simulink model "teleop_sim"  (R2019a)
settings: Solver=VariableStepAuto  StartTime=0.0  StopTime=10  MaxStep=dt  RelTol=1e-3
model workspace: external: MATLAB File .\teleop_sim_setup.m (data not in the file)
undefined symbols (not defined in the file): A_v, b, d_T, derivative_phases, epsilon, f_0, K_d, K_p, m, Ts, v_0, w_v, x_0
settings Model: Creator=Shane  LastModifiedBy=17stf1
settings DataIOCC: ReturnWorkspaceOutputs=off
settings DebuggingCC: PregeneratedLibrarySubsystemCodeDiagnostic=none  StrictBusMsg=WarnOnBusTreatedAsVector  ArithmeticOperatorsInVariantConditions=warning
settings SFSimCC: SimUseLocalCustomCode=off
settings RTWCC: RTWUseLocalCustomCode=off

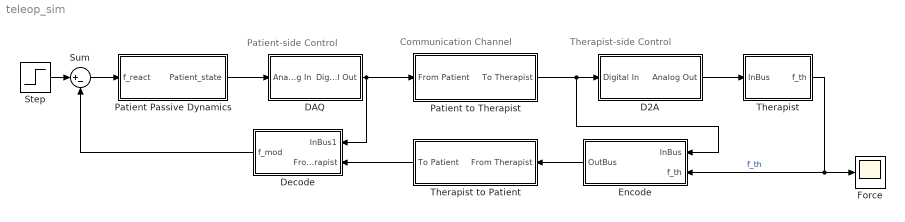
== system teleop_sim ==
  note: Patient-side Control
  note: Therapist-side Control
  note: Communication Channel
  D2A : Subsystem
  DAQ : Subsystem
  Decode : Subsystem
  Encode : Subsystem
  Force : Scope
  Patient Passive Dynamics : Subsystem
  Patient to Therapist : Subsystem
  Step : Step  After=0  SampleTime=0
  Sum : Sum  Inputs=|+-
  Therapist : Subsystem
  Therapist to Patient : Subsystem
  wires:
  Sum/1 -> Patient Passive Dynamics/1(f_react)
  Patient Passive Dynamics/1(Patient_state) -> DAQ/1(Analog In)
  Step/1 -> Sum/1
  Therapist/1(f_th) -> Force/1, Encode/2(f_th)  "f_th"
  Patient to Therapist/1(To Therapist) -> D2A/1(Digital In), Encode/1(InBus)
  Encode/1(OutBus) -> Therapist to Patient/1(From Therapist)
  Therapist to Patient/1(To Patient) -> Decode/2(FromTherapist)
  Decode/1(f_mod) -> Sum/2
  DAQ/1(Digital Out) -> Decode/1(InBus1), Patient to Therapist/1(From Patient)
  D2A/1(Analog Out) -> Therapist/1(InBus)

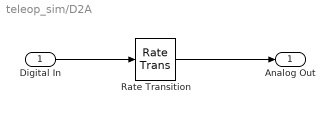
== system teleop_sim/D2A ==
  Digital In : Inport
  Rate Transition : RateTransition
  Analog Out : Outport
  wires:
  Digital In/1 -> Rate Transition/1
  Rate Transition/1 -> Analog Out/1

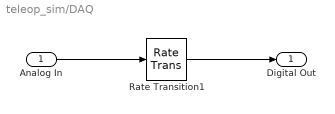
== system teleop_sim/DAQ ==
  Analog In : Inport
  Rate Transition1 : RateTransition  OutPortSampleTime=Ts
  Digital Out : Outport
  wires:
  Analog In/1 -> Rate Transition1/1
  Rate Transition1/1 -> Digital Out/1

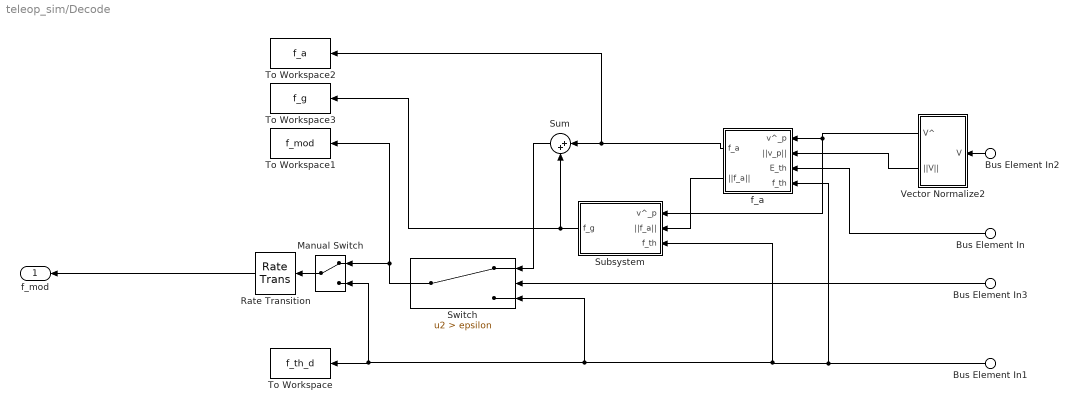
== system teleop_sim/Decode ==
  Bus Element In2 : Inport  PortName=InBus1  Element=v_p
  Bus Element In : Inport  Port=2  PortName=FromTherapist  Element=E_th
  Bus Element In1 : Inport  Port=2  PortName=FromTherapist  Element=f_th
  Bus Element In3 : Inport  Port=2  PortName=FromTherapist  Element=v_mag
  Manual Switch : ManualSwitch
  Rate Transition : RateTransition
  Subsystem : Subsystem
  Sum : Sum  Inputs=|++
  Switch : Switch  Criteria=u2 > Threshold  Threshold=epsilon
  To Workspace : ToWorkspace  VariableName=f_th_d  SaveFormat=Structure With Time  SampleTime=-1
  To Workspace1 : ToWorkspace  VariableName=f_mod  SaveFormat=Structure With Time  SampleTime=-1
  To Workspace2 : ToWorkspace  VariableName=f_a  SaveFormat=Structure With Time  SampleTime=-1
  To Workspace3 : ToWorkspace  VariableName=f_g  SaveFormat=Structure With Time  SampleTime=-1
  Vector Normalize2 : Subsystem  mask{min_magnitude=epsilon}
      mask prompts: min_magnitude "Minimum magnitude:"
  f_a : Subsystem
  f_mod : Outport
  wires:
  Sum/1 -> Switch/1
  Bus Element In2/1 -> Vector Normalize2/1(V)
  Vector Normalize2/1(V^) -> f_a/1(v^_p), Subsystem/1(v^_p)
  Manual Switch/1 -> Rate Transition/1
  Bus Element In1/1 -> f_a/4(f_th), Subsystem/3(f_th), Manual Switch/2, To Workspace/1, Switch/3
  Rate Transition/1 -> f_mod/1
  Subsystem/1(f_g) -> Sum/2, To Workspace3/1
  Bus Element In3/1 -> Switch/2
  Switch/1 -> Manual Switch/1, To Workspace1/1
  f_a/1(f_a) -> To Workspace2/1, Sum/1
  Vector Normalize2/2(||V||) -> f_a/2(||v_p||)
  Bus Element In/1 -> f_a/3(E_th)
  f_a/2(||f_a||) -> Subsystem/2(||f_a||)

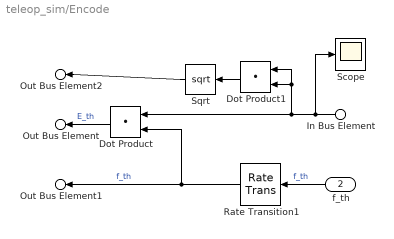
== system teleop_sim/Encode ==
  In Bus Element : Inport  PortName=InBus  Element=v_p
  f_th : Inport  Port=2
  Dot Product : DotProduct  InputSameDT=on  OutDataTypeStr=Inherit: Inherit via internal rule
  Dot Product1 : DotProduct  InputSameDT=on  OutDataTypeStr=Inherit: Inherit via internal rule
  Rate Transition1 : RateTransition  InitialCondition=f_0  OutPortSampleTime=Ts
  Scope : Scope
  Sqrt : Sqrt  SaturateOnIntegerOverflow=on
  Out Bus Element : Outport  PortName=OutBus  Element=E_th
  Out Bus Element1 : Outport  PortName=OutBus  Element=f_th
  Out Bus Element2 : Outport  PortName=OutBus  Element=v_mag
  wires:
  f_th/1 -> Rate Transition1/1  "f_th"
  Dot Product/1 -> Out Bus Element/1  "E_th"
  Rate Transition1/1 -> Dot Product/2, Out Bus Element1/1  "f_th"
  In Bus Element/1 -> Scope/1, Dot Product/1, Dot Product1/2, Dot Product1/1
  Dot Product1/1 -> Sqrt/1
  Sqrt/1 -> Out Bus Element2/1

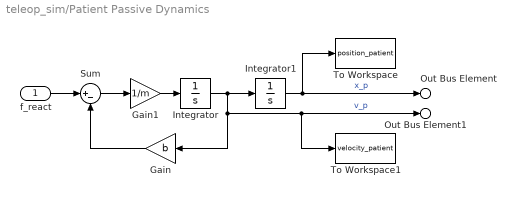
== system teleop_sim/Patient Passive Dynamics ==
  f_react : Inport
  Gain : Gain  Gain=b
  Gain1 : Gain  Gain=1/m
  Integrator : Integrator  InitialCondition=v_0
  Integrator1 : Integrator  InitialCondition=x_0
  Sum : Sum  Inputs=|+-
  To Workspace : ToWorkspace  VariableName=position_patient  SaveFormat=Structure With Time  SampleTime=Ts
  To Workspace1 : ToWorkspace  VariableName=velocity_patient  SaveFormat=Structure With Time  SampleTime=Ts
  Out Bus Element : Outport  PortName=Patient_state  Element=x_p
  Out Bus Element1 : Outport  PortName=Patient_state  Element=v_p
  wires:
  Integrator/1 -> Gain/1, Out Bus Element1/1, To Workspace1/1, Integrator1/1  "v_p"
  Integrator1/1 -> To Workspace/1, Out Bus Element/1  "x_p"
  f_react/1 -> Sum/1
  Sum/1 -> Gain1/1
  Gain/1 -> Sum/2
  Gain1/1 -> Integrator/1

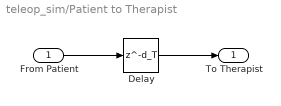
== system teleop_sim/Patient to Therapist ==
  From Patient : Inport
  Delay : Delay  DelayLength=d_T
  To Therapist : Outport
  wires:
  From Patient/1 -> Delay/1
  Delay/1 -> To Therapist/1

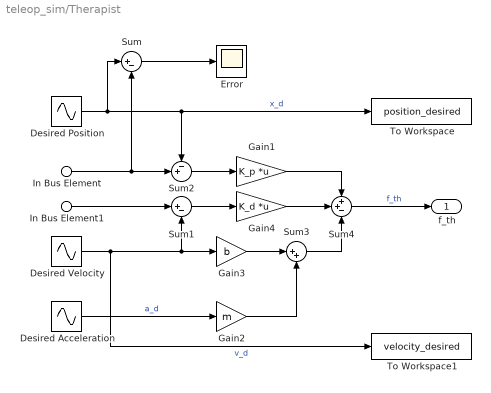
== system teleop_sim/Therapist ==
  In Bus Element1 : Inport  PortName=InBus  Element=v_p
  In Bus Element : Inport  PortName=InBus  Element=x_p
  Desired Acceleration : Sin  Amplitude=-A_v*w_v^2  Frequency=w_v  Phase=derivative_phases(:,3)  SampleTime=0
  Desired Position : Sin  Amplitude=A_v  Frequency=w_v  Phase=derivative_phases(:,1)  SampleTime=0
  Desired Velocity : Sin  Amplitude=A_v*w_v  Frequency=w_v  Phase=derivative_phases(:,2)  SampleTime=0
  Error : Scope
  Gain1 : Gain  Gain=K_p  Multiplication=Matrix(K*u)
  Gain2 : Gain  Gain=m
  Gain3 : Gain  Gain=b
  Gain4 : Gain  Gain=K_d  Multiplication=Matrix(K*u)
  Sum : Sum  Inputs=|+-
  Sum1 : Sum  Inputs=|+-
  Sum2 : Sum  Inputs=-+|
  Sum3 : Sum  Inputs=|++
  Sum4 : Sum  Inputs=++-
  To Workspace : ToWorkspace  VariableName=position_desired  SaveFormat=Structure With Time  SampleTime=Ts
  To Workspace1 : ToWorkspace  VariableName=velocity_desired  SaveFormat=Structure With Time  SampleTime=Ts
  f_th : Outport
  wires:
  Desired Position/1 -> Sum/1, Sum2/1, To Workspace/1  "x_d"
  Desired Velocity/1 -> Sum1/2, Gain3/1, To Workspace1/1  "v_d"
  Sum2/1 -> Gain1/1
  Desired Acceleration/1 -> Gain2/1  "a_d"
  Gain3/1 -> Sum3/1
  Gain2/1 -> Sum3/2
  Gain1/1 -> Sum4/1
  Sum4/1 -> f_th/1  "f_th"
  In Bus Element/1 -> Sum/2, Sum2/2
  In Bus Element1/1 -> Sum1/1
  Sum1/1 -> Gain4/1
  Sum3/1 -> Sum4/3
  Gain4/1 -> Sum4/2
  Sum/1 -> Error/1

== system teleop_sim/Therapist to Patient ==
  From Therapist : Inport
  Delay : Delay  DelayLength=d_T
  To Patient : Outport
  wires:
  From Therapist/1 -> Delay/1
  Delay/1 -> To Patient/1

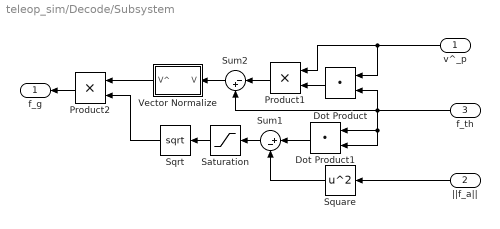
== system teleop_sim/Decode/Subsystem ==
  v^_p : Inport
  ||f_a|| : Inport  Port=2
  f_th : Inport  Port=3
  Dot Product : DotProduct  InputSameDT=on  OutDataTypeStr=Inherit: Inherit via internal rule
  Dot Product1 : DotProduct  InputSameDT=on  OutDataTypeStr=Inherit: Inherit via internal rule
  Product1 : Product
  Product2 : Product
  Saturation : Saturate  UpperLimit=inf  LowerLimit=0
  Sqrt : Sqrt  SaturateOnIntegerOverflow=on
  Square : Math  Operator=square  SaturateOnIntegerOverflow=on
  Sum1 : Sum  Inputs=|+-
  Sum2 : Sum  Inputs=|-+
  Vector Normalize : Subsystem  mask{min_magnitude=epsilon}
      mask prompts: min_magnitude "Minimum magnitude:"
  f_g : Outport
  wires:
  Sqrt/1 -> Product2/2
  f_th/1 -> Dot Product1/2, Dot Product1/1, Sum2/2, Dot Product/2
  Sum2/1 -> Vector Normalize/1(V)
  Vector Normalize/1(V^) -> Product2/1
  v^_p/1 -> Product1/1, Dot Product/1
  Product1/1 -> Sum2/1
  ||f_a||/1 -> Square/1
  Dot Product1/1 -> Sum1/1
  Dot Product/1 -> Product1/2
  Product2/1 -> f_g/1
  Sum1/1 -> Saturation/1
  Square/1 -> Sum1/2
  Saturation/1 -> Sqrt/1

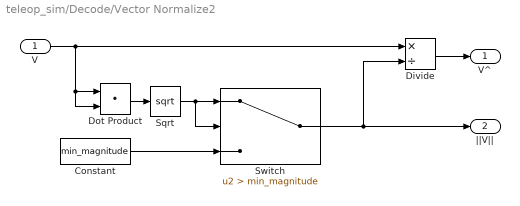
== system teleop_sim/Decode/Vector Normalize2 ==
  V : Inport
  Constant : Constant  Value=min_magnitude
  Divide : Product  Inputs=*/
  Dot Product : DotProduct  OutMin=epsilon  InputSameDT=on  OutDataTypeStr=Inherit: Inherit via internal rule
  Sqrt : Sqrt  SaturateOnIntegerOverflow=on
  Switch : Switch  Criteria=u2 > Threshold  Threshold=min_magnitude
  V^ : Outport
  ||V|| : Outport  Port=2
  wires:
  V/1 -> Divide/1, Dot Product/1, Dot Product/2
  Divide/1 -> V^/1
  Dot Product/1 -> Sqrt/1
  Switch/1 -> ||V||/1, Divide/2
  Constant/1 -> Switch/3
  Sqrt/1 -> Switch/2, Switch/1

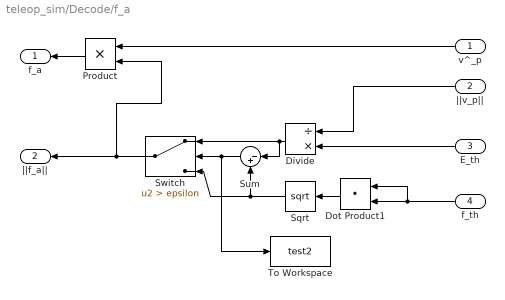
== system teleop_sim/Decode/f_a ==
  v^_p : Inport
  ||v_p|| : Inport  Port=2
  E_th : Inport  Port=3
  f_th : Inport  Port=4
  Divide : Product  Inputs=/*
  Dot Product1 : DotProduct  InputSameDT=on  OutDataTypeStr=Inherit: Inherit via internal rule
  Product : Product
  Sqrt : Sqrt  SaturateOnIntegerOverflow=on
  Sum : Sum  Inputs=|-+
  Switch : Switch  Criteria=u2 > Threshold  Threshold=epsilon
  To Workspace : ToWorkspace  VariableName=test2  SaveFormat=Timeseries  SampleTime=-1
  f_a : Outport
  ||f_a|| : Outport  Port=2
  wires:
  ||v_p||/1 -> Divide/1
  E_th/1 -> Divide/2
  Product/1 -> f_a/1
  v^_p/1 -> Product/1
  Divide/1 -> Switch/1, Sum/1
  Sum/1 -> To Workspace/1, Switch/2
  Dot Product1/1 -> Sqrt/1
  Switch/1 -> Product/2, ||f_a||/1
  f_th/1 -> Dot Product1/1, Dot Product1/2
  Sqrt/1 -> Switch/3, Sum/2

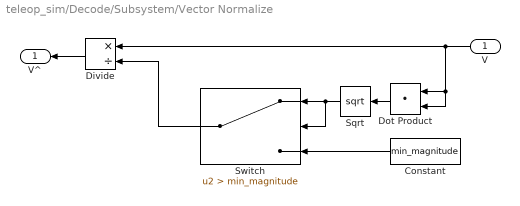
== system teleop_sim/Decode/Subsystem/Vector Normalize ==
  V : Inport
  Constant : Constant  Value=min_magnitude
  Divide : Product  Inputs=*/
  Dot Product : DotProduct  OutMin=epsilon  InputSameDT=on  OutDataTypeStr=Inherit: Inherit via internal rule
  Sqrt : Sqrt  SaturateOnIntegerOverflow=on
  Switch : Switch  Criteria=u2 > Threshold  Threshold=min_magnitude
  V^ : Outport
  wires:
  V/1 -> Dot Product/1, Dot Product/2, Divide/1
  Divide/1 -> V^/1
  Dot Product/1 -> Sqrt/1
  Switch/1 -> Divide/2
  Constant/1 -> Switch/3
  Sqrt/1 -> Switch/2, Switch/1
